simulink model "MPC_Demo_wuguzhang"  (R2024a)
settings: Solver=ode1  StartTime=0.001  StopTime=16  FixedStep=0.001  RelTol=1e-3  EnableMultiTasking=on
model workspace (MAT data in the model file):
  cc = 10
libraries: simulink x3, SignalEditorBlockLib x3, Solver_SF x1, slpidlib x1
(part 1 of 5)
settings Model: Creator=Dell  LastModifiedBy=Xiao Hu
settings SolverCC: AlgebraicLoopSolver=TrustRegion
settings OptimizationCC: LifeSpan=inf
settings DebuggingCC: MultiTaskRateTransMsg=warning  UnconnectedInputMsg=warning  UnconnectedOutputMsg=warning  UnconnectedLineMsg=warning  SFUnexpectedBacktrackingDiag=warning  SFNoUnconditionalDefaultTransitionDiag=warning  SFExecutionAtInitializationDiag=none  ArithmeticOperatorsInVariantConditions=warning
settings ModelReferenceCC: EnableRefExpFcnMdlSchedulingChecks=on
settings SFSimCC: SimUseLocalCustomCode=off  CustomCodeUndefinedFunction=UseInterfaceOnly
settings RTWCC: RTWUseLocalCustomCode=off  GPUComputeCapability=3.5
settings CodeAppCC: StateflowObjectComments=on
settings GRTTargetCC: TargetLangStandard=C89/C90 (ANSI)
settings ConfigComp: CovMetricSettings=dw  CovSaveCumulativeToWorkspaceVar=on  CovSaveSingleToWorkspaceVar=on  CovExternalEMLEnable=off

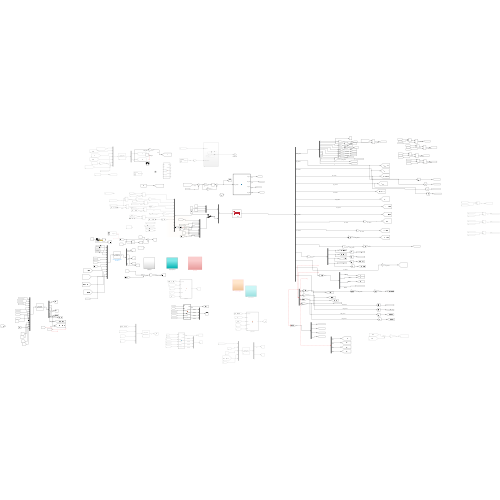
[thumbnail: Simulink's stored preview of the top-level diagram]
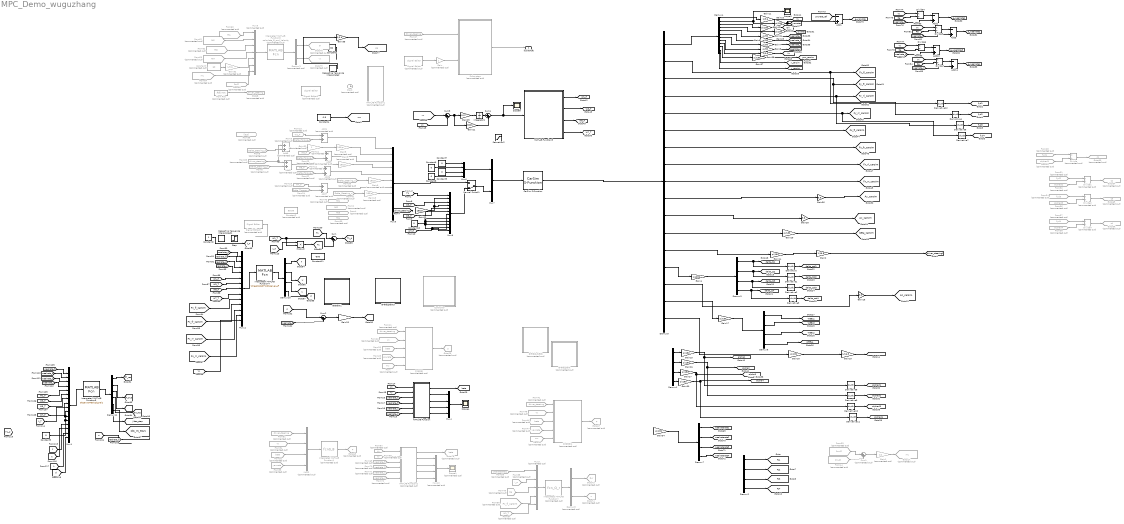
== system MPC_Demo_wuguzhang ==
  note: Product
  Add{1..3,10..11} (5 alike) : Sum  Inputs=-+
  Add{4..9} (6 alike) : Sum  Commented=on
  CarSim S-Function : Solver_SF/CarSim S-Function  Priority=1  SIMFILE=simfile.sim  Run_RTs=off  vs_state_ind=Run  StopMode_ind=Vehicle Model
  Clock : Clock  Commented=on
  Constant : Constant  Value=80
  Constant1 : Constant  Commented=on  Value=60
  Constant{5..10} (6 alike) : Constant  Value=0
  Constant11 : Constant  Value=-500
  Constant2 : Constant
  Constant3 : Constant  Commented=on  Value=89.99
  Constant4 : Constant  Value=0.8
  Controller : Subsystem  Commented=on
  Demux{1..3,6..7,10} (6 alike) : Demux
  Demux11 : Demux  Outputs=6
  Demux4 : Demux  Outputs=12
  Demux5 : Demux  Outputs=[12 1 1 1 1 1 1 1 1 1 1 1 1 4 1 4 1]
  Demux8 : Demux  Commented=on  Outputs=2
  Demux9 : Demux  Commented=on  Outputs=2
  Derivative{,1..4,6..12} (12 alike) : Derivative
  Divide{,1..3} (4 alike) : Product  Commented=on  Inputs=*/
  Divide{4..7} (4 alike) : Product  Inputs=*/
  From : From  Commented=on  GotoTag=mu  TagVisibility=global
  From File : FromFile  Commented=on  FileName=角度.mat  OutDataTypeStr=double  SampleTime=0.001
  From{11,27,41,51} (4 alike) : From  Commented=on  GotoTag=driver_steering  TagVisibility=global
  From12 : From  Commented=on  GotoTag=W5_T  TagVisibility=global
  From13 : From  Commented=on  GotoTag=W1_T  TagVisibility=global
  From2 : From  Commented=on  GotoTag=Fd2  TagVisibility=global
  From20 : From  Commented=on  GotoTag=beta  TagVisibility=global
  From21 : From  Commented=on  GotoTag=W3_T  TagVisibility=global
  From22 : From  Commented=on  GotoTag=Delta_Torque_rl  TagVisibility=global
  From23 : From  Commented=on  GotoTag=Delta_Torque_fr  TagVisibility=global
  From24 : From  Commented=on  GotoTag=Delta_Torque_rr  TagVisibility=global
  From25 : From  Commented=on  GotoTag=yawrate  TagVisibility=global
  From{26,48,54,67} (4 alike) : From  Commented=on  GotoTag=Vx  TagVisibility=global
  From28 : From  Commented=on  GotoTag=fyd1  TagVisibility=global
  From29 : From  Commented=on  GotoTag=W7_T  TagVisibility=global
  From3 : From  Commented=on  GotoTag=Delta_Torque_fl  TagVisibility=global
  From30 : From  Commented=on  GotoTag=alphad1  TagVisibility=global
  From31 : From  Commented=on  GotoTag=fyd2  TagVisibility=global
  From32 : From  Commented=on  GotoTag=alphad2  TagVisibility=global
  From33 : From  Commented=on  GotoTag=mu1  TagVisibility=global
  From34 : From  Commented=on  GotoTag=fyd3  TagVisibility=global
  From35 : From  Commented=on  GotoTag=driver_steering
  From36 : From  Commented=on  GotoTag=alphad3  TagVisibility=global
  From37 : From  Commented=on  GotoTag=fyd4  TagVisibility=global
  From38 : From  Commented=on  GotoTag=alphad4  TagVisibility=global
  From39 : From  Commented=on  GotoTag=Delta_Steering_rl  TagVisibility=global
  From4 : From  Commented=on  GotoTag=Fd3  TagVisibility=global
  From40 : From  Commented=on  GotoTag=mu  TagVisibility=global
  From42 : From  Commented=on  GotoTag=Delta_Steering_rr  TagVisibility=global
  From43 : From  Commented=on  GotoTag=Fd1  TagVisibility=global
  From44 : From  Commented=on  GotoTag=mu2  TagVisibility=global
  From46 : From  Commented=on  GotoTag=beta  TagVisibility=global
  From47 : From  Commented=on  GotoTag=yawrate  TagVisibility=global
  From49 : From  Commented=on  GotoTag=Re  TagVisibility=global
  From5 : From  Commented=on  GotoTag=Delta_Steering_fl  TagVisibility=global
  From50 : From  Commented=on  GotoTag=Fd4  TagVisibility=global
  From52 : From  Commented=on  GotoTag=beta  TagVisibility=global
  From53 : From  Commented=on  GotoTag=yawrate  TagVisibility=global
  From55 : From  Commented=on  GotoTag=I_w  TagVisibility=global
  From56 : From  Commented=on  GotoTag=Fx_fl_carsim  TagVisibility=global
  From57 : From  Commented=on  GotoTag=W1_T  TagVisibility=global
  From58 : From  Commented=on  GotoTag=last
  From59 : From  Commented=on  GotoTag=weelraterate1  TagVisibility=global
  From6 : From  Commented=on  GotoTag=Delta_Steering_fr  TagVisibility=global
  From60 : From  Commented=on  GotoTag=Fz1  TagVisibility=global
  From61 : From  Commented=on  GotoTag=Fz2  TagVisibility=global
  From62 : From  Commented=on  GotoTag=Fz3  TagVisibility=global
  From63 : From  Commented=on  GotoTag=Fz4  TagVisibility=global
  From64 : From  Commented=on  GotoTag=mu  TagVisibility=global
  From66 : From  Commented=on  GotoTag=tw1  TagVisibility=global
  From68 : From  Commented=on  GotoTag=Vy  TagVisibility=global
  From69 : From  Commented=on  GotoTag=weelrate_fl  TagVisibility=global
  From70 : From  Commented=on  GotoTag=weelrate_fr  TagVisibility=global
  From71 : From  Commented=on  GotoTag=weelrate_rl  TagVisibility=global
  From72 : From  Commented=on  GotoTag=weelrate_rr  TagVisibility=global
  Gain : Gain  Commented=on
  Gain1 : Gain  Commented=on  Gain=1/2
  Gain{10,12,14..15,17..18,23,26..27,29..30,34,37} (13 alike) : Gain  Gain=pi/180
  Gain11 : Gain  Gain=1/3.6
  Gain{3,5,9,13} (4 alike) : Gain  Commented=on  Gain=180/pi
  Gain16 : Gain  Gain=9.8
  Gain19 : Gain  Gain=1/16.8
  Gain2 : Gain  Gain=1/16.8
  Gain20 : Gain  Gain=1.5/0.005
  Gain21 : Gain  Gain=5000
  Gain22 : Gain  Gain=180/pi
  Gain{6..8,24} (4 alike) : Gain  Gain=pi/30
  Gain25 : Gain  Gain=0.07
  Gain28 : Gain  Gain=9.8
  Gain32 : Gain  Commented=on  Gain=1/3.6
  Gain35 : Gain  Gain=1/3.6
  Gain36 : Gain  Gain=9.8
  Gain38 : Gain  Gain=1/3.6
  Gain39 : Gain  Commented=on
  Gain4 : Gain  Gain=1/1000
  Goto17 : Goto  Commented=on  GotoTag=mu  TagVisibility=global
  Goto28 : Goto  Commented=on  GotoTag=p  TagVisibility=global
  Goto59 : Goto  Commented=on  GotoTag=c1  TagVisibility=global
  Goto64 : Goto  Commented=on  GotoTag=c2  TagVisibility=global
  Goto65 : Goto  Commented=on  GotoTag=c3  TagVisibility=global
  Goto66 : Goto  Commented=on  GotoTag=c4  TagVisibility=global
  Goto67 : Goto  Commented=on  GotoTag=p  TagVisibility=global
  Goto68 : Goto  Commented=on  GotoTag=p  TagVisibility=global
  Goto73 : Goto  Commented=on  GotoTag=Q_r  TagVisibility=global
  Goto74 : Goto  Commented=on  GotoTag=n  TagVisibility=global
  Goto75 : Goto  Commented=on  GotoTag=vx  TagVisibility=global
  Goto76 : Goto  Commented=on  GotoTag=G  TagVisibility=global
  Goto78 : Goto  Commented=on  GotoTag=beta  TagVisibility=global
  Goto8 : Goto  Commented=on  GotoTag=driver_steering  TagVisibility=global
  Integrator1 : Integrator
  Interpreted MATLAB Function1 : MATLABFcn  Commented=on  MATLABFcn=fcn0_8  OutputDimensions=1  Output1D=off
  Interpreted MATLAB Function2 : MATLABFcn  Commented=on  MATLABFcn=fcn_Q_r  OutputDimensions=2  Output1D=off
  Interpreted MATLAB Function3 : MATLABFcn  Commented=on  MATLABFcn=calculate_G_and_Velocity  OutputDimensions=2  Output1D=off
  Interpreted MATLAB Function4 : MATLABFcn  MATLABFcn=WheelRotASTWObserver_LF  OutputDimensions=4  Output1D=off
  Interpreted MATLAB Function5 : MATLABFcn  MATLABFcn=ObserverMetricSignals  OutputDimensions=6  Output1D=off
  MATLAB Function : MATLAB Function  TreatAsAtomicUnit=on
  MATLAB Function1 : MATLAB Function  Commented=on  TreatAsAtomicUnit=on
  MATLAB Function2 : MATLAB Function  Commented=on  TreatAsAtomicUnit=on
  MATLAB Function5 : MATLAB Function  TreatAsAtomicUnit=on
  Manual Switch1 : ManualSwitch  CurrentSetting=0
  Mux1 : Mux  Inputs=16
  Mux10 : Mux  Commented=on
  Mux11 : Mux  Inputs=13
  Mux2 : Mux  Commented=on
  Mux3 : Mux  Commented=on  Inputs=5
  Mux4 : Mux
  Mux5 : Mux  Inputs=12
  Mux6 : Mux
  Mux7 : Mux  Inputs=[4,12]
  Mux8 : Mux  Inputs=12
  Mux9 : Mux  Commented=on  Inputs=7
  Product : Product
  Repeating Sequence Interpolated : simulink/Sources/Repeating Sequence Interpolated  OutValues=[60.76 83.52 41].'  TimeValues=[0 8.5 16].'  LookUpMeth=Interpolation-Use End Values  tsamp=0.001  OutMin=[]  OutMax=[]  OutDataTypeStr=double  OutputDataTypeScalingMode=double  OutDataType=fixdt(0,8)  OutScaling=2^-10
  Repeating Sequence Interpolated1 : simulink/Sources/Repeating Sequence Interpolated  OutValues=[1 1 0.2 0.2].'  TimeValues=[0 3 3.01 16].'  LookUpMeth=Interpolation-Use End Values  tsamp=0.001  OutMin=[]  OutMax=[]  OutDataTypeStr=double  OutputDataTypeScalingMode=double  OutDataType=fixdt(0,8)  OutScaling=2^-10
  Saturation2 : Saturate  UpperLimit=6400  LowerLimit=-6400
  Scope1 : Scope  Commented=on
  Scope3 : Scope
  Scope4 : Scope
  Scope8 : Scope
  Signal Editor : SignalEditorBlockLib/Signal Editor  Commented=on  FileName=Tdist.mat  ActiveScenario=Scenario  ActiveSignal=Signal 1  IsBus=off  OutputBusObjectStr=Bus: BusObject  SampleTime=0  Interpolate=off  ZeroCross=off  OutputAfterFinalValue=Setting to zero  Unit=inherit  PreserveSignalName=on  ApplySigPropsToAllScenarios=on  ApplySigPropsToAllSignals=off
  Signal Editor1 : SignalEditorBlockLib/Signal Editor  Commented=on  FileName=untitled111.mat  ActiveScenario=Scenario  ActiveSignal=Signal 1  IsBus=off  OutputBusObjectStr=Bus: BusObject  SampleTime=0  Interpolate=off  ZeroCross=off  OutputAfterFinalValue=Holding final value  Unit=inherit  PreserveSignalName=on  ApplySigPropsToAllScenarios=on  ApplySigPropsToAllSignals=off
  Signal Editor2 : SignalEditorBlockLib/Signal Editor  Commented=on  FileName=Tdist.mat  ActiveScenario=Scenario  ActiveSignal=Signal 1  IsBus=off  OutputBusObjectStr=Bus: BusObject  SampleTime=0  Interpolate=off  ZeroCross=off  OutputAfterFinalValue=Setting to zero  Unit=inherit  PreserveSignalName=on  ApplySigPropsToAllScenarios=on  ApplySigPropsToAllSignals=off
  Step : Step  Time=4  Before=1  After=-1  SampleTime=0
  Subsystem : Subsystem  Commented=on
  Sum : Sum  Inputs=|+-
  Sum1 : Sum  Commented=on  Inputs=|++
  Sum2 : Sum  Inputs=|-+
  Sum3 : Sum  Inputs=|+-
  Sum4 : Sum  Inputs=|++
  区域判断 : MATLAB Function  Commented=on  TreatAsAtomicUnit=on
  区域判断1 : MATLAB Function  Commented=on  TreatAsAtomicUnit=on
  参数模块1 : Subsystem
  参考值生成模块 : Subsystem  Commented=on
  参考模型模块 : Subsystem  Commented=on
  参考模型模块3 : Subsystem
  实际转向角 : Outport
  tag scope: Ax_carsim=global, Ay_carsim=global, Az_carsim=global, Fx_fl_carsim=global, Fx_fr_carsim=global, Fx_rl_carsim=global, Fx_rr_carsim=global, Fy_fl_carsim=global, Fy_fr_carsim=global, Fy_rl_carsim=global, Fy_rr_carsim=global, Fz1=global, Fz2=global, Fz3=global, Fz4=global, T1=global, T1_d=global, Vx=global, Vy=global, W1_T=global, W3_T=global, W5_T=global, W7_T=global, WEEL1=global, WEEL2=global, WEEL3=global, WEEL4=global, alpha1=global, alpha2=global, alpha3=global, alpha4=global, alphad1=global, alphad2=global, alphad3=global, alphad4=global, beta=global, beta_carsim=global, d=global, d_model=global, delta_zs1=global, delta_zs2=global, delta_zs3=global, delta_zs4=global, delta_zsd1=global, delta_zsd2=global, delta_zsd3=global, delta_zsd4=global, driver_steering10=global, driver_steering5=global, e_weelrate1=global, e_weelrate2=global, e_weelrate3=global, e_weelrate4=global, e_yawrate=global, err_res=global, err_true=global, f=global, fT_res=global, fT_true=global, fyd1=global, fyd2=global, fyd3=global, fyd4=global, jitter_step=global, k=global, k_T=global, mu=global, obs_inj_equiv=global, roll=global, rollrate=global, vx=global, w=global, weelrate_fl=global, weelrate_fr=global, weelrate_rl=global, weelrate_rr=global, weelraterate1=global, weelraterate2=global, weelraterate3=global, weelraterate4=global, x_carsim=global, y_carsim=global, yaw_carsim=global, yawrate=global
  wires:
  [Vx] -> MATLAB Function/1(Vx)
  [Vy] -> MATLAB Function/2(Vy)
  [weelrate_fl] -> MATLAB Function/3(omega_1)
  [weelrate_fr] -> MATLAB Function/4(omega_2)
  [weelrate_rl] -> MATLAB Function/5(omega_3)
  [weelrate_rr] -> MATLAB Function/6(omega_4)
  MATLAB Function/2(lamda1) -> Mux4/1  "lamda1"
  MATLAB Function/3(lamda2) -> Mux4/2  "lamda2"
  MATLAB Function/4(lamda3) -> Mux4/3  "lamda3"
  MATLAB Function/5(lamda4) -> Mux4/4  "lamda4"
  Mux4/1 -> Scope4/1
  MATLAB Function/1(beta) -> [beta]  "beta"
  Gain23/1 -> [rollrate]  "rollrate"
  Demux4/2 -> Scope3/1, Gain10/1
  Gain36/1 -> [Ay_carsim]  "Ay_carsim"
  Demux5/4 -> Derivative6/1, [Fy_rl_carsim]  "Fyrl_carsim"
  Demux4/8 -> Gain8/1
  Demux5/8 -> [Fx_rl_carsim]  "Fzrl_carsim"
  Demux4/12 -> [y_carsim]  "Y"
  Gain28/1 -> [Ax_carsim]  "Ax_carsim"
  Gain29/1 -> [beta_carsim]  "beta_carsim"
  Demux4/10 -> Gain37/1
  Gain37/1 -> [yaw_carsim]  "yaw_carsim"
  Demux4/9 -> Gain38/1
  Gain38/1 -> [Vx]  "vx_carsim"
  Demux5/1 -> Demux4/1  "delta_carsim"
  Demux5/3 -> Derivative4/1, [Fy_fr_carsim]  "Fyfr_carsim"
  Demux4/3 -> Gain12/1
  Demux4/1 -> Gain11/1
  Gain12/1 -> [roll]  "roll"
  Gain10/1 -> Add1/2, [yawrate]  "yawrate"
  Gain8/1 -> [weelrate_rr]  "weelrate4"
  Demux5/9 -> [Fx_rr_carsim]  "Fzrr_carsim"
  Gain11/1 -> [Vy]  "Vy"
  Demux4/5 -> Gain24/1
  Demux4/6 -> Gain6/1
  Gain7/1 -> [weelrate_rl]  "weelrate3"
  Gain6/1 -> [weelrate_fr]  "weelrate2"
  Gain24/1 -> [weelrate_fl]  "轮速实际值"
  Demux5/11 -> Gain28/1  "w_rl_carsim"
  Demux4/4 -> Gain23/1
  Demux5/5 -> Derivative7/1, [Fy_rr_carsim]  "Fyrr_carsim"
  Demux4/7 -> Gain7/1
  Demux5/2 -> Derivative12/1, [Fy_fl_carsim]  "Fyfl_carsim"
  Demux5/6 -> [Fx_fl_carsim]  "Fzfl_carsim"
  Demux5/10 -> Gain36/1  "Ay_carsim"
  Demux4/11 -> [x_carsim]  "X"
  Demux5/12 -> Gain29/1
  Demux5/7 -> [Fx_fr_carsim]  "Fzfr_carsim"
  CarSim S-Function/1 -> Demux5/1
  Demux5/13 -> Gain14/1
  Gain2/1 -> [driver_steering5]  "ds"
  ? -> Demux2/1
  Demux2/1 -> [Fz1]  "mu1"
  Demux2/2 -> [Fz2]  "mu2"
  Demux2/3 -> [Fz3]  "mu3"
  Demux2/4 -> [Fz4]  "mu4"
  From33/1 -> Sum1/1
  From44/1 -> Sum1/2
  Sum1/1 -> Gain1/1
  Gain1/1 -> Goto17/1  "ds"
  Constant4/1 -> [mu]
  Demux5/14 -> Gain4/1
  Demux3/1 -> Derivative/1, [delta_zs1]
  Demux3/2 -> Derivative1/1, [delta_zs2]
  Demux3/3 -> Derivative2/1, [delta_zs3]
  Demux3/4 -> Derivative3/1, [delta_zs4]
  Derivative/1 -> [delta_zsd1]
  Derivative1/1 -> [delta_zsd2]
  Derivative2/1 -> [delta_zsd3]
  Derivative3/1 -> [delta_zsd4]
  Gain4/1 -> Demux3/1
  Gain21/1 -> Sum4/2
  MATLAB Function5/2(Tor_R1) -> [W3_T]  "T_R1"
  Sum3/1 -> Gain25/1, Gain21/1
  Sum4/1 -> Scope8/1, MATLAB Function5/1(Drive_torque)
  MATLAB Function5/4(Tor_R2) -> [W7_T]  "T_R2"
  [vx] -> Sum3/1  "Vx_d"
  Integrator1/1 -> Sum4/1
  Gain25/1 -> Integrator1/1
  [Vx] -> Sum3/2  "vx"
  MATLAB Function5/1(Tor_L1) -> [W1_T]  "T_L1"
  MATLAB Function5/3(Tor_L2) -> [W5_T]  "T_L2"
  From6/1 -> Add8/2  "delta3"
  From39/1 -> Gain9/1
  From5/1 -> Add9/2
  Add8/1 -> Gain3/1  "总的转角2"
  Constant7/1 -> Mux6/1
  Constant9/1 -> Mux6/3
  From35/1 -> Add9/1, Add8/1
  Add6/1 -> Mux5/5  "T3"
  Mux8/1 -> Manual Switch1/2  "u"
  From22/1 -> Add6/2  "delta3"
  Mux7/1 -> CarSim S-Function/1  "u"
  From13/1 -> Add4/1
  Constant6/1 -> Mux6/2
  From23/1 -> Add5/2  "delta2"
  From24/1 -> Add7/2
  From3/1 -> Add4/2  "delta1"
  [driver_steering] -> ?
  Mux5/1 -> Manual Switch1/1  "u"
  Mux6/1 -> Mux7/1  "u"
  Constant8/1 -> Mux6/4
  From21/1 -> Add5/1
  From29/1 -> Add7/1  "delta4"
  [W7_T] -> Mux8/7  "q1"
  [W3_T] -> Mux8/3  "q1"
  Constant10/1 -> Mux8/12, Mux8/11, Mux8/10, Mux8/6, Mux8/8, Mux8/9
  From File/1 -> Goto8/1
  From12/1 -> Add6/1
  From42/1 -> Gain13/1
  Gain14/1 -> Gain2/1  "beta_carsim"
  Demux5/15 -> Gain16/1  "w_rl_carsim"
  Gain16/1 -> [Az_carsim]  "Ax_carsim"
  Demux6/2 -> [WEEL3]  "WEEL3"
  Demux6/4 -> [WEEL4]  "WEEL4"
  Demux6/3 -> [WEEL2]  "WEEL2"
  Demux5/16 -> Gain17/1
  Demux6/1 -> [WEEL1]  "WEEL1"
  Gain17/1 -> Demux6/1
  Manual Switch1/1 -> Mux7/2  "add_Mz"
  Demux5/17 -> Gain18/1
  Gain18/1 -> Gain19/1  "beta_carsim"
  Gain19/1 -> [driver_steering10]  "ds1"
  From11/1 -> 区域判断/1(sw_angle)
  区域判断/1(p) -> Goto28/1  "p"
  From26/1 -> 区域判断/2(Vx)
  From/1 -> 区域判断/5(miu)
  From25/1 -> 区域判断/4(gamma)
  From20/1 -> 区域判断/3(beta)
  Subsystem/1(实际转向角) -> 实际转向角/1
  Gain/1 -> Subsystem/2(外部扰动力矩)
  Signal Editor/1 -> Gain/1  "Tdist"
  From27/1 -> Subsystem/1(期望转向)
  Signal Editor2/1 -> ?  "Tdist"
  Gain22/1 -> Mux8/2, Mux8/4
  Derivative7/1 -> [fyd4]
  Derivative6/1 -> [fyd3]
  Derivative12/1 -> [fyd1]
  Demux1/1 -> Gain15/1  "Fyfl_carsim"
  Derivative11/1 -> [alphad4]
  Demux1/4 -> Gain30/1  "Fyrr_carsim"
  Derivative8/1 -> [alphad1]
  Demux1/3 -> Gain27/1  "Fyrl_carsim"
  Derivative9/1 -> [alphad2]
  Demux1/2 -> Gain26/1  "Fyfr_carsim"
  Derivative10/1 -> [alphad3]
  ? -> Demux1/1
  From28/1 -> Divide/1
  From30/1 -> Divide/2
  Divide/1 -> Goto59/1  "c1"
  From31/1 -> Divide1/1
  Divide1/1 -> Goto64/1  "c2"
  From32/1 -> Divide1/2
  From34/1 -> Divide2/1
  Divide2/1 -> Goto65/1  "c3"
  From36/1 -> Divide2/2
  From38/1 -> Divide3/2
  Divide3/1 -> Goto66/1
  From37/1 -> Divide3/1
  Gain15/1 -> Derivative8/1, [alpha1]  "beta_carsim"
  Gain26/1 -> Derivative9/1, [alpha2]  "beta_carsim"
  Gain27/1 -> Derivative10/1, [alpha3]  "beta_carsim"
  Gain30/1 -> Derivative11/1, [alpha4]  "beta_carsim"
  Derivative4/1 -> [fyd2]
  From48/1 -> 区域判断1/2(Vx)
  区域判断1/1(p) -> Goto67/1  "p"
  From46/1 -> 区域判断1/3(beta)
  From41/1 -> 区域判断1/1(sw_angle)
  From47/1 -> 区域判断1/4(gamma)
  From40/1 -> 区域判断1/5(miu)
  From54/1 -> Mux2/2
  From52/1 -> Mux2/3
  From51/1 -> Mux2/1
  From53/1 -> Mux2/4
  Mux2/1 -> Interpreted MATLAB Function1/1
  Interpreted MATLAB Function1/1 -> Goto68/1  "p"
  Gain5/1 -> Mux5/2
  Add5/1 -> Mux5/3  "T2"
  Gain3/1 -> Mux5/4
  Gain9/1 -> Mux5/6
  Add7/1 -> Mux5/7  "T4"
  Gain13/1 -> Mux5/8
  Demux7/3 -> [weelraterate3]
  Demux7/1 -> [weelraterate1]
  Demux7/2 -> [weelraterate2]
  Demux7/4 -> [weelraterate4]
  Gain34/1 -> Demux7/1
  ? -> Gain34/1
  From59/1 -> Mux3/1
  From55/1 -> Mux3/2
  From49/1 -> Mux3/3
  From56/1 -> Mux3/4
  Mux3/1 -> Interpreted MATLAB Function2/1
  From57/1 -> Mux3/5
  Demux8/1 -> Goto73/1  "Q_r"
  Interpreted MATLAB Function2/1 -> Demux8/1
  Demux8/2 -> Goto74/1  "n"
  From62/1 -> Mux9/3
  From63/1 -> Mux9/4
  From60/1 -> Mux9/1
  Mux9/1 -> Interpreted MATLAB Function3/1
  From61/1 -> Mux9/2
  Constant1/1 -> Gain32/1
  Interpreted MATLAB Function3/1 -> Demux9/1  "p"
  Demux9/2 -> Goto75/1  "vx"
  Demux9/1 -> Goto76/1
  From64/1 -> Mux9/6  "Vx_d"
  Gain32/1 -> Mux9/5  "Vx_d"
  From66/1 -> Mux9/7
  Gain35/1 -> [vx]  "vx_d"
  Repeating Sequence Interpolated/1 -> Gain35/1  "theta_des"
  From72/1 -> MATLAB Function2/6(omega_4)
  MATLAB Function2/2(lamda1) -> Mux10/1  "lamda1"
  MATLAB Function2/3(lamda2) -> Mux10/2  "lamda2"
  MATLAB Function2/5(lamda4) -> Mux10/4  "lamda4"
  From71/1 -> MATLAB Function2/5(omega_3)
  MATLAB Function2/4(lamda3) -> Mux10/3  "lamda3"
  From70/1 -> MATLAB Function2/4(omega_2)
  MATLAB Function2/1(beta) -> Goto78/1  "beta"
  Mux10/1 -> Scope1/1
  From68/1 -> MATLAB Function2/2(Vy)
  From67/1 -> MATLAB Function2/1(Vx)
  From69/1 -> MATLAB Function2/3(omega_1)
  [yawrate_ref] -> Add1/1
  Add1/1 -> [e_yawrate]  "e_yawrate"
  [Vx] -> Divide4/1
  [Re] -> Divide4/2
  Divide4/1 -> Add2/1  "c1"
  [weelrate_fl] -> Add2/2
  Divide5/1 -> Add3/1  "c1"
  [Re] -> Divide5/2
  [weelrate_fr] -> Add3/2
  [Vx] -> Divide5/1
  [Re] -> Divide6/2
  [Vx] -> Divide6/1
  [weelrate_rr] -> Add11/2
  Divide7/1 -> Add11/1  "c1"
  Divide6/1 -> Add10/1  "c1"
  [Re] -> Divide7/2
  [Vx] -> Divide7/1
  [weelrate_rl] -> Add10/2
  Add2/1 -> [e_weelrate1]  "e_weelrate1"
  Add3/1 -> [e_weelrate2]  "e_weelrate2"
  Add10/1 -> [e_weelrate3]  "e_weelrate3"
  Add11/1 -> [e_weelrate4]  "e_weelrate4"
  Add4/1 -> Mux5/1  "T1"
  Add9/1 -> Gain39/1  "总的转角1"
  Gain39/1 -> Gain5/1
  Mux11/1 -> Interpreted MATLAB Function4/1
  [weelrate_fl] -> Mux11/1
  [weelrate_fr] -> Mux11/2
  [weelrate_rl] -> Mux11/3
  [weelrate_rr] -> Mux11/4
  [W1_T] -> Mux11/5
  [W3_T] -> Mux11/6
  [W5_T] -> Mux11/7
  [W7_T] -> Mux11/8
  [Fx_fl_carsim] -> Mux11/9
  [Fx_fr_carsim] -> Mux11/10
  [Fx_rr_carsim] -> Mux11/11
  [Fx_rr_carsim] -> Mux11/12
  Interpreted MATLAB Function4/1 -> Demux10/1  "p"
  Demux10/3 -> [k]  "k"
  Demux10/2 -> [w]  "轮速估计值"
  Demux10/4 -> [d]  "d"
  Demux10/1 -> [f]  "未知输入估计值"
  [Vx] -> Mux11/13
  [T1] -> Mux8/1
  [W1_T] -> Sum/2, Product/2
  Product/1 -> [T1]
  [T1] -> Sum/1
  Sum/1 -> [T1_d]
  Sum2/1 -> Gain20/1  "d_model"
  [w] -> Sum2/1
  [weelrate_fl] -> Sum2/2
  Gain20/1 -> [d_model]  "未知输入实际值"
  [W5_T] -> Mux8/5
  Constant2/1 -> [k_T]
  [w] -> ?
  [weelrate_fl] -> ?
  Demux11/4 -> [err_res]  "err_res"
  Demux11/1 -> [fT_res]  "fT_res"
  [W5_T] -> Mux1/7
  Interpreted MATLAB Function5/1 -> Demux11/1  "p"
  Mux1/1 -> Interpreted MATLAB Function5/1
  [W7_T] -> Mux1/8
  [W1_T] -> Mux1/5
  [weelrate_fr] -> Mux1/2
  [weelrate_rr] -> Mux1/4
  Demux11/3 -> [err_true]  "err_true"
  [W3_T] -> Mux1/6
  [weelrate_rl] -> Mux1/3
  [weelrate_fl] -> Mux1/1
  Demux11/2 -> [fT_true]  "fT_true"
  [k_T] -> Product/1
  [k_T] -> Mux1/9
  Constant5/1 -> Mux1/11, Mux1/10, Mux1/12
  [f] -> Mux1/13
  [w] -> Mux1/14
  [k] -> Mux1/15
  [d] -> Mux1/16
  Demux11/5 -> [jitter_step]  "jitter_step"
  Demux11/6 -> [obs_inj_equiv]  "obs_inj_equiv"
  Constant/1 -> ?  "theta_des"

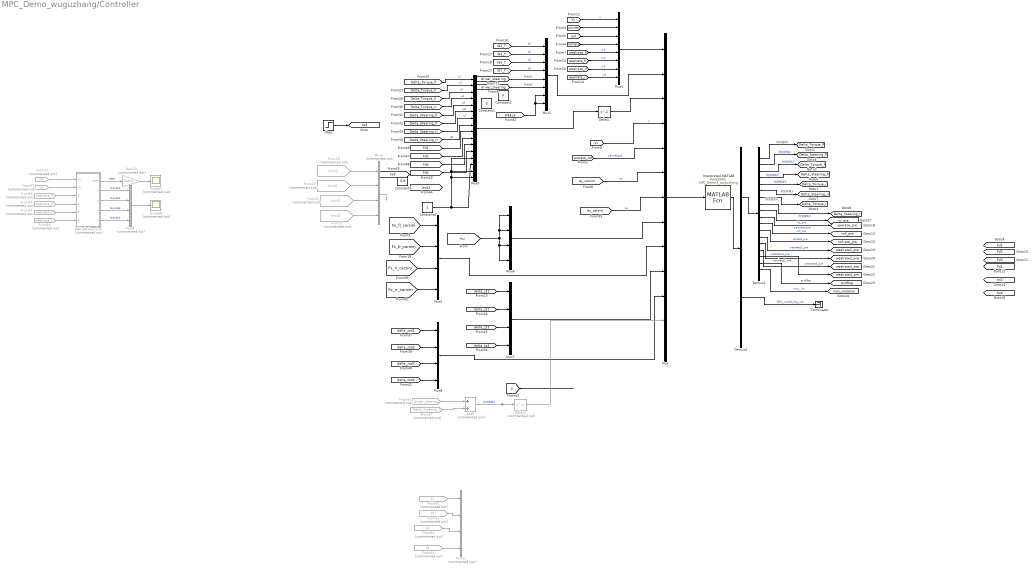
== system MPC_Demo_wuguzhang/Controller ==
  Add9 : Sum  Commented=on
  Constant1 : Constant  Value=0
  Constant2 : Constant  Value=0
  Constant3 : Constant  Value=0.8
  Constant4 : Constant
  Delay1 : Delay  DelayLength=1  InitialCondition=0
  Delay2 : Delay  Commented=on  DelayLength=1  InitialCondition=0
  Demux1 : Demux  Outputs=18
  Demux2 : Demux  Outputs=[18,481]
  From19 : From  Commented=on  GotoTag=mu1  TagVisibility=global
  From20 : From  Commented=on  GotoTag=mu2  TagVisibility=global
  From21 : From  Commented=on  GotoTag=mu3  TagVisibility=global
  From22 : From  Commented=on  GotoTag=mu4  TagVisibility=global
  From50 : From  Commented=on  GotoTag=driver_steering  TagVisibility=global
  From51 : From  Commented=on  GotoTag=Vx  TagVisibility=global
  From52 : From  Commented=on  GotoTag=Vy  TagVisibility=global
  From53 : From  Commented=on  GotoTag=weelrate_fl  TagVisibility=global
  From54 : From  Commented=on  GotoTag=weelrate_fr  TagVisibility=global
  From55 : From  Commented=on  GotoTag=weelrate_rl  TagVisibility=global
  From56 : From  Commented=on  GotoTag=weelrate_rr  TagVisibility=global
  From57 : From  Commented=on  GotoTag=Delta_Steering_fl  TagVisibility=global
  From60 : From  Commented=on  GotoTag=c1  TagVisibility=global
  From61 : From  Commented=on  GotoTag=c2  TagVisibility=global
  From62 : From  Commented=on  GotoTag=c3  TagVisibility=global
  From63 : From  Commented=on  GotoTag=c4  TagVisibility=global
  Gain15 : Gain  Commented=on  Gain=180/pi
  Interpreted MATLAB Function1 : MATLABFcn  MATLABFcn=MPC_Demo3_wuguzhang  OutputDimensions=499  Output1D=off
  MATLAB Function : MATLAB Function  Commented=on  TreatAsAtomicUnit=on
  Mux : Mux  Inputs=[8,8,16,1,1,1,1,4,4,4,4,1,1]
  Mux1 : Mux  Inputs=8
  Mux12 : Mux  Commented=on
  Mux2 : Mux  Inputs=8
  Mux3 : Mux  Inputs=16
  Mux4 : Mux  Commented=on
  Mux{5..8} (4 alike) : Mux
  Mux9 : Mux  Commented=on
  Scope1 : Scope  Commented=on
  Scope4 : Scope  Commented=on
  Step : Step  Time=3  Before=1  After=0  SampleTime=0
  Terminator : Terminator
  tag scope: Delta_Steering_fl=global, Delta_Steering_fr=global, Delta_Steering_rl=global, Delta_Steering_rr=global, Delta_Torque_fl=global, Delta_Torque_fr=global, Delta_Torque_rl=global, Delta_Torque_rr=global, Fd1=global, Fd2=global, Fd3=global, Fd4=global, exitflag=global, max_violation=global, roll_pre=global, rollrate_pre=global, tw2=global, tw3=global, tw4=global, vy_pre=global, weelrate1_pre=global, weelrate2_pre=global, weelrate3_pre=global, weelrate4_pre=global, yawrate_pre=global
  wires:
  [Vy] -> Mux1/1  "v"
  [yawrate] -> Mux1/2
  [roll] -> Mux1/3
  [rollrate] -> Mux1/4
  [weelrate_fl] -> Mux1/5  "w1"
  [weelrate_fr] -> Mux1/6  "w2"
  [weelrate_rl] -> Mux1/7  "w3"
  [weelrate_rr] -> Mux1/8  "w4"
  [W7_T] -> Mux2/4  "q4"
  [W5_T] -> Mux2/3  "q3"
  [W3_T] -> Mux2/2  "q2"
  [W1_T] -> Mux2/1  "q1"
  [Delta_Steering_fl] -> Mux3/5  "u5"
  [Delta_Steering_rl] -> Mux3/7  "u7"
  [Delta_Torque_rr] -> Mux3/4  "u4"
  [Delta_Torque_fr] -> Mux3/2  "u2"
  [Delta_Steering_fr] -> Mux3/6  "u6"
  [Delta_Torque_fl] -> Mux3/1  "u1"
  [Delta_Steering_rr] -> Mux3/8  "u8"
  [Delta_Torque_rl] -> Mux3/3  "u3"
  Mux3/1 -> Delay1/1
  Interpreted MATLAB Function1/1 -> Demux2/1
  Demux1/8 -> [Delta_Steering_rr]  "附加转角4"
  Demux1/1 -> [Delta_Torque_fl]  "附加扭矩1"
  Mux1/1 -> Mux/1
  Mux2/1 -> Mux/2
  Delay1/1 -> Mux/3
  [Vx] -> Mux/4  "u"
  Demux1/2 -> [Delta_Steering_fl]  "附加转角1"
  Demux1/4 -> [Delta_Steering_fr]  "附加转角2"
  Demux1/5 -> [Delta_Torque_rl]  "附加扭矩3"
  Demux1/6 -> [Delta_Steering_rl]  "附加转角3"
  Demux1/7 -> [Delta_Torque_rr]  "附加扭矩4"
  Mux/1 -> Interpreted MATLAB Function1/1
  [yawrate_ref] -> Mux/5  "yawrate_d"
  [Ay_carsim] -> Mux/6  "ay"
  [Ax_carsim] -> Mux/7  "ax"
  Mux4/1 -> ?
  [driver_steering] -> Mux2/6  "theta2"
  [Fx_fl_carsim] -> Mux5/1
  [Fx_fr_carsim] -> Mux5/2
  [Fx_rl_carsim] -> Mux5/3
  [Fx_rr_carsim] -> Mux5/4
  Mux5/1 -> Mux/9
  From19/1 -> Mux4/1
  From20/1 -> Mux4/2
  From21/1 -> Mux4/3
  From22/1 -> Mux4/4
  [mu] -> Mux6/2, Mux6/1, Mux6/4, Mux6/3
  Mux6/1 -> Mux/8
  Mux7/1 -> Mux/10
  [delta_zs1] -> Mux7/1
  [delta_zs2] -> Mux7/2
  [delta_zs3] -> Mux7/3
  [delta_zs4] -> Mux7/4
  [delta_zsd4] -> Mux8/4
  [delta_zsd2] -> Mux8/2
  [delta_zsd1] -> Mux8/1
  [delta_zsd3] -> Mux8/3
  Mux8/1 -> Mux/11
  ? -> [Fd1]  "fd1"
  ? -> [Fd2]  "fd2"
  ? -> [Fd3]  "fd3"
  ? -> [Fd4]  "fd4"
  [Fd4] -> Mux3/12
  [Fd3] -> Mux3/11
  [Fd2] -> Mux3/10
  [Fd1] -> Mux3/9
  Demux1/3 -> [Delta_Torque_fr]  "附加扭矩2"
  ? -> ?
  ? -> [tw2]
  ? -> ?
  ? -> [tw4]
  Constant4/1 -> Mux3/16, Mux3/15, Mux3/13, Mux3/14
  MATLAB Function/2(lamda1) -> Mux9/1  "lamda1"
  From56/1 -> MATLAB Function/6(omega_4)
  From53/1 -> MATLAB Function/3(omega_1)
  MATLAB Function/1(beta) -> Gain15/1  "beta"
  MATLAB Function/5(lamda4) -> Mux9/4  "lamda4"
  From51/1 -> MATLAB Function/1(Vx)
  From52/1 -> MATLAB Function/2(Vy)
  Mux9/1 -> Scope4/1
  From55/1 -> MATLAB Function/5(omega_3)
  MATLAB Function/4(lamda3) -> Mux9/3  "lamda3"
  MATLAB Function/3(lamda2) -> Mux9/2  "lamda2"
  From54/1 -> MATLAB Function/4(omega_2)
  Gain15/1 -> Scope1/1
  From60/1 -> Mux12/1
  From61/1 -> Mux12/2
  From62/1 -> Mux12/3
  From63/1 -> Mux12/4
  [p] -> ?
  Demux1/9 -> [vy_pre]  "Vy_pre"
  Add9/1 -> Delay2/1  "总的转角1"
  From57/1 -> Add9/2
  From50/1 -> Add9/1
  Delay2/1 -> Mux/12
  Demux1/10 -> [yawrate_pre]  "yawrate_pre"
  Step/1 -> [tw3]
  [WEEL3] -> Mux2/8, Mux2/7
  Demux1/11 -> [roll_pre]  "roll_pre"
  Demux1/12 -> [rollrate_pre]  "rollrate_pre"
  Demux1/13 -> [weelrate1_pre]  "weelrate1_pre"
  Demux1/14 -> [weelrate2_pre]  "weelrate2_pre"
  Demux1/15 -> [weelrate3_pre]  "weelrate3_pre"
  Demux1/16 -> [weelrate4_pre]  "weelrate4_pre"
  [driver_steering] -> Mux2/5  "theta1"
  Demux1/17 -> [exitflag]  "exitflag"
  Demux1/18 -> [max_violation]  "max_vio"
  Demux2/1 -> Demux1/1
  Demux2/2 -> Terminator/1  "MPC_model_log_vec"

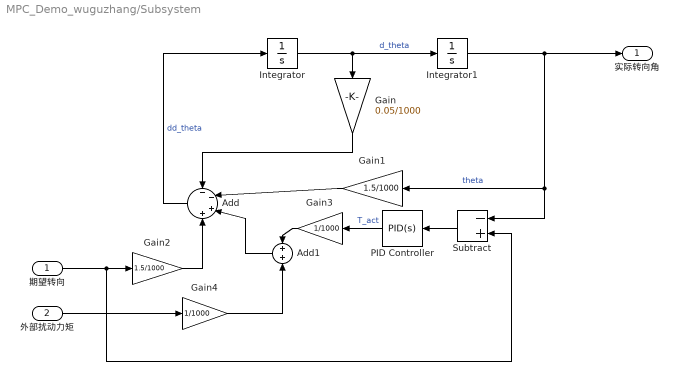
== system MPC_Demo_wuguzhang/Subsystem ==
  期望转向 : Inport
  外部扰动力矩 : Inport  Port=2
  Add : Sum  Inputs=--++
  Add1 : Sum
  Gain : Gain  Gain=0.05/1000
  Gain1 : Gain  Gain=1.5/1000
  Gain2 : Gain  Gain=1.5/1000
  Gain3 : Gain  Gain=1/1000
  Gain4 : Gain  Gain=1/1000
  Integrator : Integrator
  Integrator1 : Integrator
  PID Controller : slpidlib/PID Controller  Controller=PID  Form=Parallel  TimeDomain=Continuous-time  UseExternalTs=off  SampleTime=-1  IntegratorMethod=Forward Euler  FilterMethod=Forward Euler  ControllerParametersSource=internal  P=10000  I=100  UseKiTs=off  D=0  UseExternalDerivativeSource=off  N=100  UseFilter=on  TunerSelectOption=Transfer Function Based (PID Tuner App)  InitialConditionSource=internal  InitialConditionForIntegrator=0  InitialConditionForFilter=0  DifferentiatorICPrevScaledInput=0  ExternalReset=none  TrackingMode=off  Kt=1  LimitOutput=off  SatLimitsSource=internal  UpperSaturationLimit=inf  LowerSaturationLimit=-inf  LinearizeAsGain=on  AntiWindupMode=none  Kb=1  LimitIntegrator=off  UpperIntegratorSaturationLimit=inf  LowerIntegratorSaturationLimit=-inf  POutMin=[]  POutMax=[]  IOutMin=[]  IOutMax=[]  DOutMin=[]  DOutMax=[]  NOutMin=[]  NOutMax=[]  SumOutMin=[]  SumOutMax=[]  SaturationOutMin=[]  SaturationOutMax=[]  PParamMin=[]  PParamMax=[]  IParamMin=[]  IParamMax=[]  DParamMin=[]  DParamMax=[]  NParamMin=[]  NParamMax=[]  KbParamMin=[]  KbParamMax=[]  KtParamMin=[]  KtParamMax=[]  KbOutMin=[]  KbOutMax=[]  KtOutMin=[]  KtOutMax=[]  IntegratorOutMin=[]  IntegratorOutMax=[]  FilterOutMin=[]  FilterOutMax=[]  SumI1OutMin=[]  SumI1OutMax=[]  SumI2OutMin=[]  SumI2OutMax=[]  SumI3OutMin=[]  SumI3OutMax=[]  SumI4OutMin=[]  SumI4OutMax=[]  SumDOutMin=[]  SumDOutMax=[]  DifferentiatorOutMin=[]  DifferentiatorOutMax=[]  FilterDiffOutCoefMin=[]  FilterDiffOutCoefMax=[]  ReciprocalOutMin=[]  ReciprocalOutMax=[]  SumDenOutMin=[]  SumDenOutMax=[]  SumNumOutMin=[]  SumNumOutMax=[]  DivideOutMin=[]  DivideOutMax=[]  UdiffTsProdOutMin=[]  UdiffTsProdOutMax=[]  NTsProdOutMin=[]  NTsProdOutMax=[]  UintegralTsProdOutMin=[]  UintegralTsProdOutMax=[]  UngainTsProdOutMin=[]  UngainTsProdOutMax=[]  ClampingZeroOutDataTypeStr=Inherit: Inherit via back propagation  ClampingZeroOutMin=[]  ClampingZeroOutMax=[]  FilterDenConstantOutDataTypeStr=Inherit: Inherit via back propagation  FilterDenConstantOutMin=[]  FilterDenConstantOutMax=[]  PCopyOutDataTypeStr=Inherit: Inherit via back propagation  PCopyOutMin=[]  PCopyOutMax=[]  NCopyOutDataTypeStr=Inherit: Inherit via back propagation  NCopyOutMin=[]  NCopyOutMax=[]  IntegratorContinuousStateAttributes=''  IntegratorStateMustResolveToSignalObject=off  IntegratorRTWStateStorageClass=Auto  FilterContinuousStateAttributes=''  FilterStateMustResolveToSignalObject=off  FilterRTWStateStorageClass=Auto  ParallelPVariant=InternalParameters  IdealPVariant=Disabled  IVariant=InternalParameters  DVariant=InternalParameters  IntegratorVariant=Continuous  SatVariant=Disabled  AWVariant=Passthrough  PCopyVariant=Disabled  TRVariant=Disabled  FdbkBlocksVariant=Forward  IdealPFdbkVariant=Disabled  SatFdbkVariant=Disabled  DerivativeFilterVariant=ContFilter  NVariant=InternalParameters  NCopyVariant=Disabled  FilterICVariant=InternalICsFilter  IntegratorICVariant=InternalICs  ExternalResetVariant=Disabled  TRSumVariant=Passthrough  SumFdbkVariant=Disabled  SumVariant=Sum_PID  TsampFilterVariant=InternalTs  TsampNgainVariant=Passthrough  TsampIntegralVariant=Disabled_SignalSpec  ExternalSaturationOutDataTypeStr=Inherit: Same as second input  DerivativeSourceVariant=ErrorSignal
  Subtract : Sum  Inputs=-+
  实际转向角 : Outport
  wires:
  期望转向/1 -> Subtract/2, Gain2/1
  Gain4/1 -> Add1/2
  Integrator/1 -> Integrator1/1, Gain/1  "d_theta"
  Integrator1/1 -> 实际转向角/1, Subtract/1, Gain1/1  "theta"
  外部扰动力矩/1 -> Gain4/1
  Subtract/1 -> PID Controller/1
  Gain3/1 -> Add1/1
  Gain2/1 -> Add/4
  Add1/1 -> Add/3
  Add/1 -> Integrator/1  "dd_theta"
  Gain/1 -> Add/1
  PID Controller/1 -> Gain3/1  "T_act"
  Gain1/1 -> Add/2

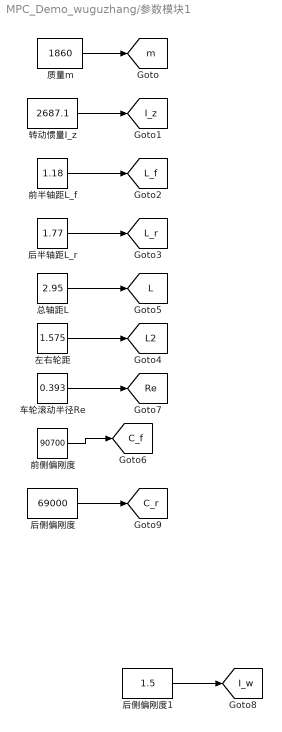
== system MPC_Demo_wuguzhang/参数模块1 ==
  前侧偏刚度 : Constant  Value=90700
  前半轴距L_f : Constant  Value=1.18
  后侧偏刚度 : Constant  Value=69000
  后侧偏刚度1 : Constant  Value=1.5
  后半轴距L_r : Constant  Value=1.77
  左右轮距 : Constant  Value=1.575
  总轴距L : Constant  Value=2.95
  质量m : Constant  Value=1860
  车轮滚动半径Re : Constant  Value=0.393
  转动惯量I_z : Constant  Value=2687.1
  tag scope: C_f=global, C_r=global, I_w=global, I_z=global, L2=global, L=global, L_f=global, L_r=global, Re=global, m=global
  wires:
  后半轴距L_r/1 -> [L_r]
  总轴距L/1 -> [L]
  车轮滚动半径Re/1 -> [Re]
  前半轴距L_f/1 -> [L_f]
  左右轮距/1 -> [L2]
  质量m/1 -> [m]
  转动惯量I_z/1 -> [I_z]
  后侧偏刚度/1 -> [C_r]
  前侧偏刚度/1 -> [C_f]
  后侧偏刚度1/1 -> [I_w]

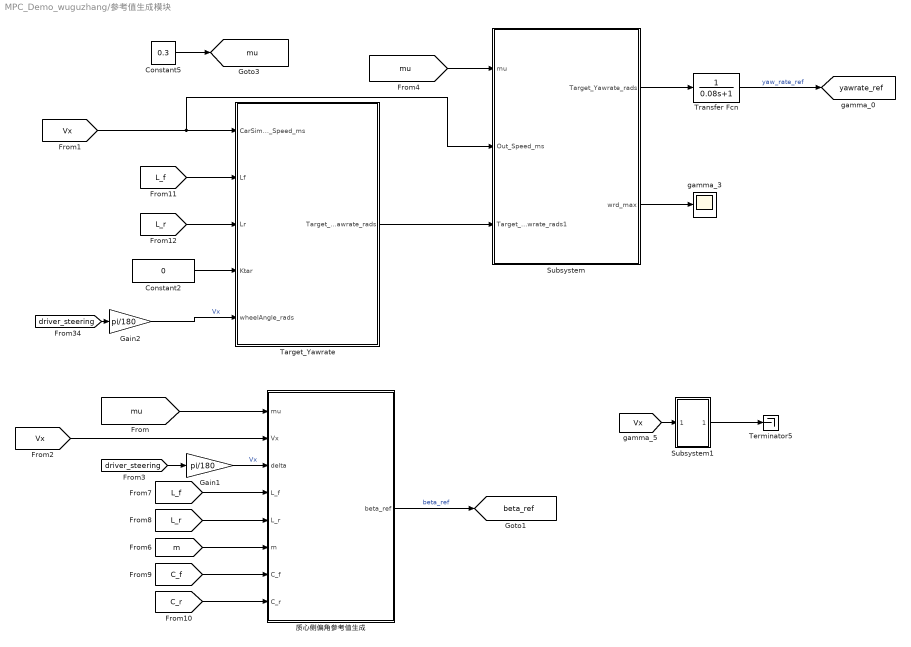
== system MPC_Demo_wuguzhang/参考值生成模块 ==
  Constant2 : Constant  Value=0
  Constant5 : Constant  Value=0.3
  Gain1 : Gain  Gain=pi/180
  Gain2 : Gain  Gain=pi/180
  Subsystem : Subsystem
  Subsystem1 : Subsystem
  Target_Yawrate : Subsystem
  Terminator5 : Terminator
  Transfer Fcn : TransferFcn  Denominator=[0.08 1]
  gamma_3 : Scope
  质心侧偏角参考值生成 : MATLAB Function  TreatAsAtomicUnit=on
  tag scope: beta_ref=global, mu=global, yawrate_ref=global
  wires:
  Target_Yawrate/1(Target_Yawrate_rads) -> Subsystem/3(Target_Yawrate_rads1)
  Subsystem/2(wrd_max) -> gamma_3/1
  [Vx] -> Subsystem/2(Out_Speed_ms), Target_Yawrate/1(CarSimOut_Speed_ms)
  [L_f] -> Target_Yawrate/2(Lf)
  [L_r] -> Target_Yawrate/3(Lr)
  [driver_steering] -> Gain2/1
  Constant2/1 -> Target_Yawrate/4(Ktar)
  Subsystem/1(Target_Yawrate_rads) -> Transfer Fcn/1
  Transfer Fcn/1 -> [yawrate_ref]  "yaw_rate_ref"
  [Vx] -> 质心侧偏角参考值生成/2(Vx)
  [driver_steering] -> Gain1/1
  质心侧偏角参考值生成/1(beta_ref) -> [beta_ref]  "beta_ref"
  [mu] -> Subsystem/1(mu)
  [mu] -> 质心侧偏角参考值生成/1(mu)
  [Vx] -> Subsystem1/1(In1)
  Subsystem1/1(Out1) -> Terminator5/1
  [m] -> 质心侧偏角参考值生成/6(m)
  [L_f] -> 质心侧偏角参考值生成/4(L_f)
  [L_r] -> 质心侧偏角参考值生成/5(L_r)
  [C_f] -> 质心侧偏角参考值生成/7(C_f)
  [C_r] -> 质心侧偏角参考值生成/8(C_r)
  Constant5/1 -> [mu]
  Gain1/1 -> 质心侧偏角参考值生成/3(delta)  "Vx"
  Gain2/1 -> Target_Yawrate/5(wheelAngle_rads)  "Vx"

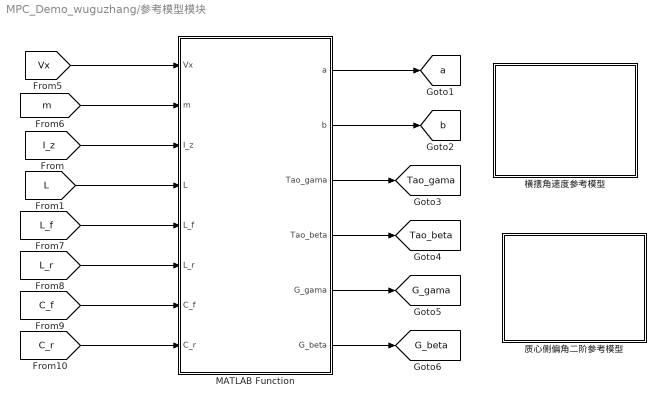
== system MPC_Demo_wuguzhang/参考模型模块 ==
  MATLAB Function : MATLAB Function  TreatAsAtomicUnit=on
  横摆角速度参考模型 : Subsystem
  质心侧偏角二阶参考模型 : Subsystem
  tag scope: G_beta=global, G_gama=global, Tao_beta=global, Tao_gama=global, a=global, b=global
  wires:
  [Vx] -> MATLAB Function/1(Vx)
  MATLAB Function/1(a) -> [a]
  MATLAB Function/2(b) -> [b]
  MATLAB Function/3(Tao_gama) -> [Tao_gama]
  MATLAB Function/4(Tao_beta) -> [Tao_beta]
  MATLAB Function/5(G_gama) -> [G_gama]
  MATLAB Function/6(G_beta) -> [G_beta]
  [m] -> MATLAB Function/2(m)
  [L_f] -> MATLAB Function/5(L_f)
  [L_r] -> MATLAB Function/6(L_r)
  [C_f] -> MATLAB Function/7(C_f)
  [C_r] -> MATLAB Function/8(C_r)
  [I_z] -> MATLAB Function/3(I_z)
  [L] -> MATLAB Function/4(L)

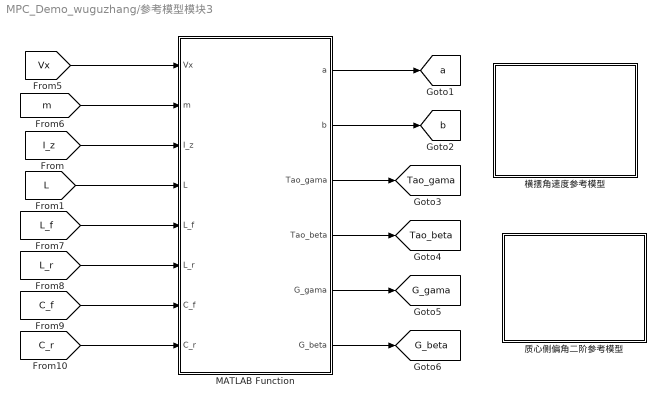
== system MPC_Demo_wuguzhang/参考模型模块3 ==
  MATLAB Function : MATLAB Function  TreatAsAtomicUnit=on
  横摆角速度参考模型 : Subsystem
  质心侧偏角二阶参考模型 : Subsystem
  tag scope: G_beta=global, G_gama=global, Tao_beta=global, Tao_gama=global, a=global, b=global
  wires:
  [Vx] -> MATLAB Function/1(Vx)
  MATLAB Function/1(a) -> [a]
  MATLAB Function/2(b) -> [b]
  MATLAB Function/3(Tao_gama) -> [Tao_gama]
  MATLAB Function/4(Tao_beta) -> [Tao_beta]
  MATLAB Function/5(G_gama) -> [G_gama]
  MATLAB Function/6(G_beta) -> [G_beta]
  [m] -> MATLAB Function/2(m)
  [L_f] -> MATLAB Function/5(L_f)
  [L_r] -> MATLAB Function/6(L_r)
  [C_f] -> MATLAB Function/7(C_f)
  [C_r] -> MATLAB Function/8(C_r)
  [I_z] -> MATLAB Function/3(I_z)
  [L] -> MATLAB Function/4(L)

== system MPC_Demo_wuguzhang/参考值生成模块/Subsystem ==
  mu : Inport
  Out_Speed_ms : Inport  Port=2
  Target_Yawrate_rads1 : Inport  Port=3
  MATLAB Function : MATLAB Function  TreatAsAtomicUnit=on
  Target_Yawrate_rads : Outport
  wrd_max : Outport  Port=2
  wires:
  Out_Speed_ms/1 -> MATLAB Function/2(vx)
  MATLAB Function/2(wrd) -> Target_Yawrate_rads/1
  mu/1 -> MATLAB Function/1(mu)
  MATLAB Function/1(wrd_max) -> wrd_max/1
  Target_Yawrate_rads1/1 -> MATLAB Function/3(wrd1)

== system MPC_Demo_wuguzhang/参考值生成模块/Subsystem1 ==
  In1 : Inport
  Constant : Constant  Value=0.01
  Ramp : simulink/Sources/Ramp  slope=1  start=0  InitialOutput=0
  Switch : Switch  Threshold=0.01  SaturateOnIntegerOverflow=off  InputSameDT=off
  Out1 : Outport
  wires:
  Switch/1 -> Out1/1
  Constant/1 -> Switch/3
  In1/1 -> Switch/1
  Ramp/1 -> Switch/2

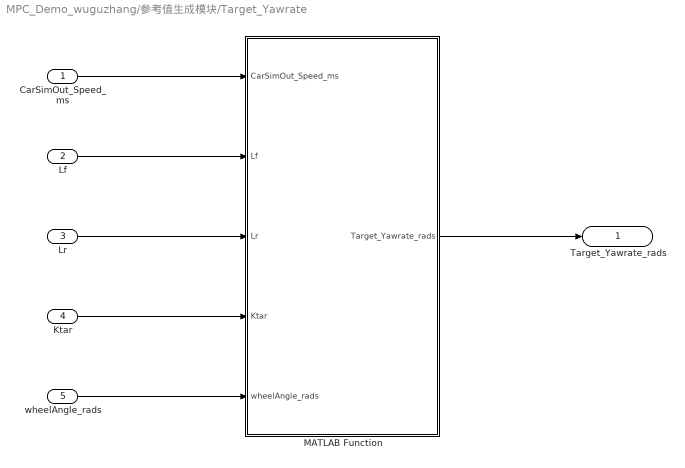
== system MPC_Demo_wuguzhang/参考值生成模块/Target_Yawrate ==
  CarSimOut_Speed_ms : Inport
  Lf : Inport  Port=2
  Lr : Inport  Port=3
  Ktar : Inport  Port=4
  wheelAngle_rads : Inport  Port=5
  MATLAB Function : MATLAB Function  TreatAsAtomicUnit=on
  Target_Yawrate_rads : Outport
  wires:
  CarSimOut_Speed_ms/1 -> MATLAB Function/1(CarSimOut_Speed_ms)
  Lf/1 -> MATLAB Function/2(Lf)
  Lr/1 -> MATLAB Function/3(Lr)
  Ktar/1 -> MATLAB Function/4(Ktar)
  wheelAngle_rads/1 -> MATLAB Function/5(wheelAngle_rads)
  MATLAB Function/1(Target_Yawrate_rads) -> Target_Yawrate_rads/1

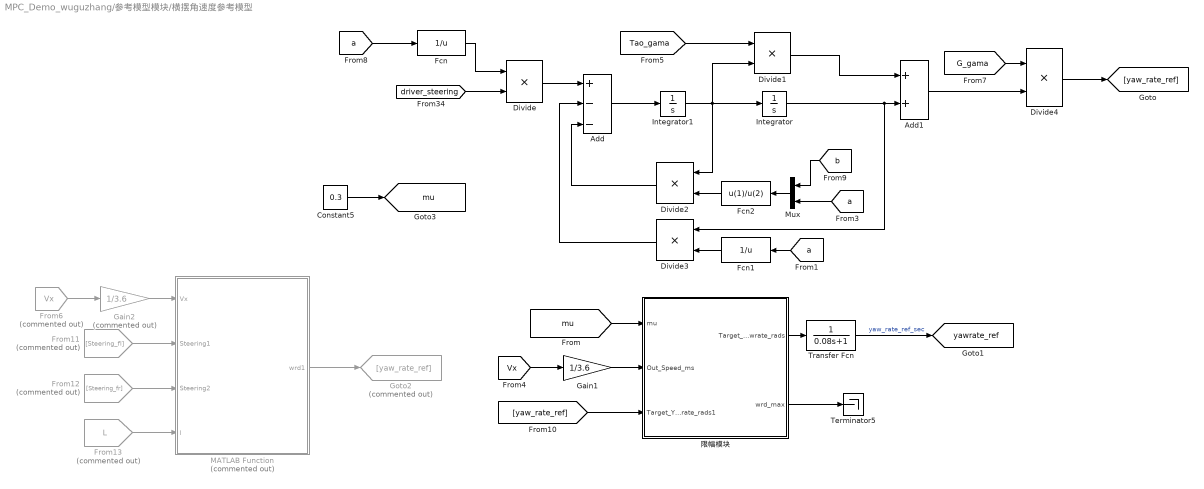
== system MPC_Demo_wuguzhang/参考模型模块/横摆角速度参考模型 ==
  Add : Sum  Inputs=+--
  Add1 : Sum
  Constant5 : Constant  Value=0.3
  Divide{,1..4} (5 alike) : Product  Inputs=**
  Fcn : Fcn  Expr=1/u
  Fcn1 : Fcn  Expr=1/u
  Fcn2 : Fcn  Expr=u(1)/u(2)
  From11 : From  Commented=on  GotoTag=Steering_fl  TagVisibility=global
  From12 : From  Commented=on  GotoTag=Steering_fr  TagVisibility=global
  From13 : From  Commented=on  GotoTag=L  TagVisibility=global
  From6 : From  Commented=on  GotoTag=Vx  TagVisibility=global
  Gain1 : Gain  Gain=1/3.6
  Gain2 : Gain  Commented=on  Gain=1/3.6
  Goto2 : Goto  Commented=on  GotoTag=yaw_rate_ref
  Integrator : Integrator
  Integrator1 : Integrator
  MATLAB Function : MATLAB Function  Commented=on  TreatAsAtomicUnit=on
  Mux : Mux  Inputs=2
  Terminator5 : Terminator
  Transfer Fcn : TransferFcn  Denominator=[0.08 1]
  限幅模块 : Subsystem
  tag scope: mu=global, yawrate_ref=global
  wires:
  Integrator/1 -> Divide3/1, Add1/2
  [G_gama] -> Divide4/1
  Add1/1 -> Divide4/2
  [Tao_gama] -> Divide1/1
  Fcn/1 -> Divide/1
  Divide4/1 -> [yaw_rate_ref]
  Fcn1/1 -> Divide3/2
  Divide2/1 -> Add/3
  Divide3/1 -> Add/2
  Fcn2/1 -> Divide2/2
  Divide/1 -> Add/1
  Divide1/1 -> Add1/1
  Integrator1/1 -> Divide2/1, Divide1/2, Integrator/1
  [driver_steering] -> Divide/2
  [a] -> Fcn/1
  [a] -> Fcn1/1
  Mux/1 -> Fcn2/1
  [b] -> Mux/1
  [a] -> Mux/2
  [mu] -> 限幅模块/1(mu)
  [Vx] -> Gain1/1
  Gain1/1 -> 限幅模块/2(Out_Speed_ms)
  [yaw_rate_ref] -> 限幅模块/3(Target_Yawrate_rads1)
  限幅模块/1(Target_Yawrate_rads) -> Transfer Fcn/1
  Transfer Fcn/1 -> [yawrate_ref]  "yaw_rate_ref_sec"
  限幅模块/2(wrd_max) -> Terminator5/1
  MATLAB Function/1(wrd1) -> Goto2/1
  From11/1 -> MATLAB Function/2(Steering1)
  From12/1 -> MATLAB Function/3(Steering2)
  From13/1 -> MATLAB Function/4(l)
  From6/1 -> Gain2/1
  Gain2/1 -> MATLAB Function/1(Vx)
  Constant5/1 -> [mu]
  Add/1 -> Integrator1/1

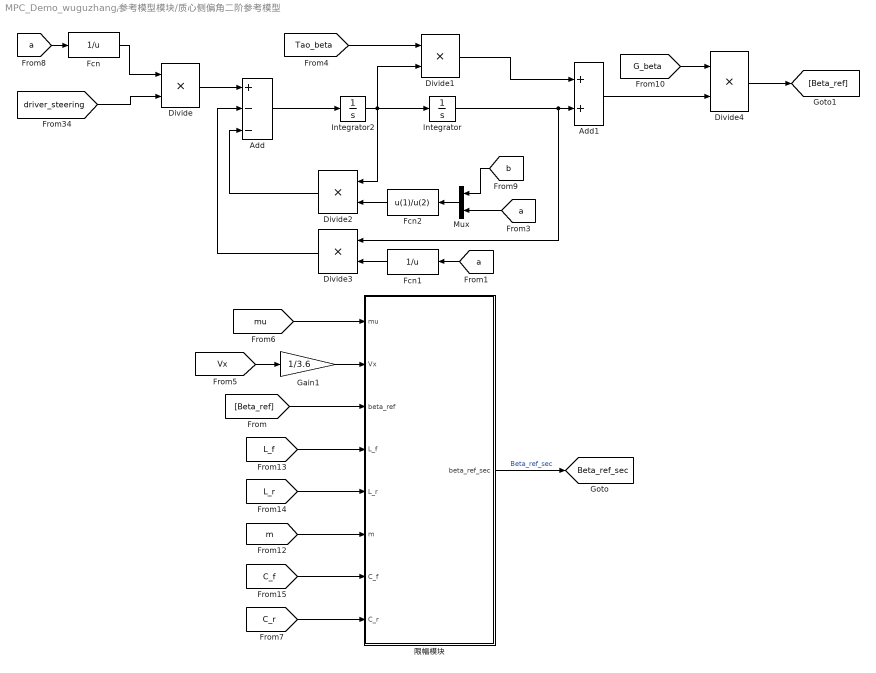
== system MPC_Demo_wuguzhang/参考模型模块/质心侧偏角二阶参考模型 ==
  Add : Sum  Inputs=+--
  Add1 : Sum
  Divide{,1..4} (5 alike) : Product  Inputs=**
  Fcn : Fcn  Expr=1/u
  Fcn1 : Fcn  Expr=1/u
  Fcn2 : Fcn  Expr=u(1)/u(2)
  Gain1 : Gain  Gain=1/3.6
  Integrator : Integrator
  Integrator2 : Integrator
  Mux : Mux  Inputs=2
  限幅模块 : MATLAB Function  TreatAsAtomicUnit=on
  tag scope: Beta_ref_sec=global
  wires:
  [a] -> Mux/2
  [b] -> Mux/1
  Mux/1 -> Fcn2/1
  [a] -> Fcn1/1
  [a] -> Fcn/1
  [driver_steering] -> Divide/2
  Integrator2/1 -> Integrator/1, Divide1/2, Divide2/1
  Divide1/1 -> Add1/1
  Divide/1 -> Add/1
  Fcn2/1 -> Divide2/2
  Divide3/1 -> Add/2
  Divide2/1 -> Add/3
  Fcn1/1 -> Divide3/2
  Divide4/1 -> [Beta_ref]
  Fcn/1 -> Divide/1
  [Tao_beta] -> Divide1/1
  Add1/1 -> Divide4/2
  [G_beta] -> Divide4/1
  Integrator/1 -> Add1/2, Divide3/1
  [mu] -> 限幅模块/1(mu)
  限幅模块/1(beta_ref_sec) -> [Beta_ref_sec]  "Beta_ref_sec"
  [Beta_ref] -> 限幅模块/3(beta_ref)
  [Vx] -> Gain1/1
  Gain1/1 -> 限幅模块/2(Vx)
  Add/1 -> Integrator2/1
  [m] -> 限幅模块/6(m)
  [L_f] -> 限幅模块/4(L_f)
  [L_r] -> 限幅模块/5(L_r)
  [C_f] -> 限幅模块/7(C_f)
  [C_r] -> 限幅模块/8(C_r)

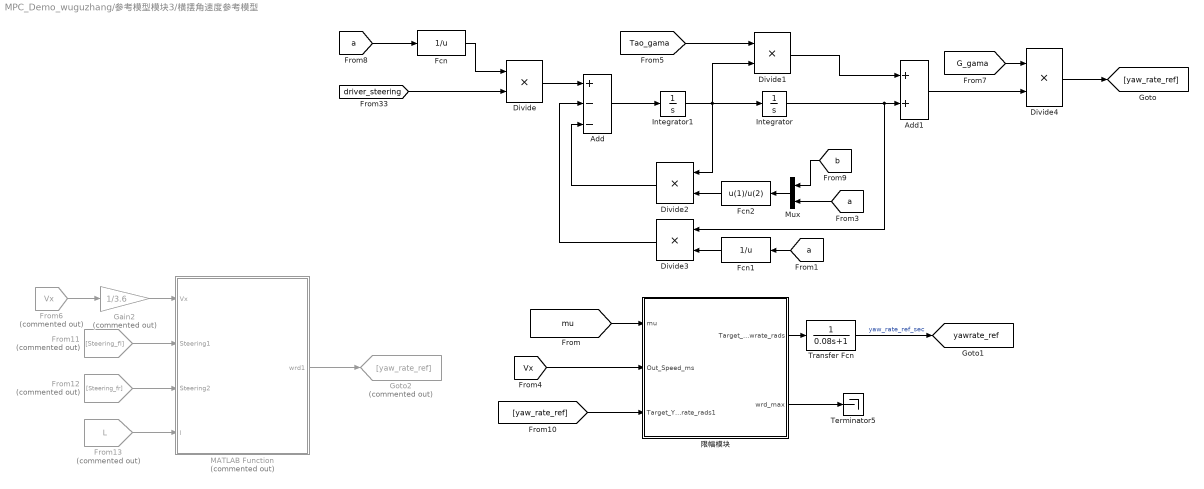
== system MPC_Demo_wuguzhang/参考模型模块3/横摆角速度参考模型 ==
  Add : Sum  Inputs=+--
  Add1 : Sum
  Divide{,1..4} (5 alike) : Product  Inputs=**
  Fcn : Fcn  Expr=1/u
  Fcn1 : Fcn  Expr=1/u
  Fcn2 : Fcn  Expr=u(1)/u(2)
  From11 : From  Commented=on  GotoTag=Steering_fl  TagVisibility=global
  From12 : From  Commented=on  GotoTag=Steering_fr  TagVisibility=global
  From13 : From  Commented=on  GotoTag=L  TagVisibility=global
  From6 : From  Commented=on  GotoTag=Vx  TagVisibility=global
  Gain2 : Gain  Commented=on  Gain=1/3.6
  Goto2 : Goto  Commented=on  GotoTag=yaw_rate_ref
  Integrator : Integrator
  Integrator1 : Integrator
  MATLAB Function : MATLAB Function  Commented=on  TreatAsAtomicUnit=on
  Mux : Mux  Inputs=2
  Terminator5 : Terminator
  Transfer Fcn : TransferFcn  Denominator=[0.08 1]
  限幅模块 : Subsystem
  tag scope: yawrate_ref=global
  wires:
  Integrator/1 -> Divide3/1, Add1/2
  [G_gama] -> Divide4/1
  Add1/1 -> Divide4/2
  [Tao_gama] -> Divide1/1
  Fcn/1 -> Divide/1
  Divide4/1 -> [yaw_rate_ref]
  Fcn1/1 -> Divide3/2
  Divide2/1 -> Add/3
  Divide3/1 -> Add/2
  Fcn2/1 -> Divide2/2
  Divide/1 -> Add/1
  Divide1/1 -> Add1/1
  Integrator1/1 -> Divide2/1, Divide1/2, Integrator/1
  [a] -> Fcn/1
  [a] -> Fcn1/1
  Mux/1 -> Fcn2/1
  [b] -> Mux/1
  [a] -> Mux/2
  [mu] -> 限幅模块/1(mu)
  [Vx] -> 限幅模块/2(Out_Speed_ms)
  [yaw_rate_ref] -> 限幅模块/3(Target_Yawrate_rads1)
  限幅模块/1(Target_Yawrate_rads) -> Transfer Fcn/1
  Transfer Fcn/1 -> [yawrate_ref]  "yaw_rate_ref_sec"
  限幅模块/2(wrd_max) -> Terminator5/1
  MATLAB Function/1(wrd1) -> Goto2/1
  From11/1 -> MATLAB Function/2(Steering1)
  From12/1 -> MATLAB Function/3(Steering2)
  From13/1 -> MATLAB Function/4(l)
  From6/1 -> Gain2/1
  Gain2/1 -> MATLAB Function/1(Vx)
  Add/1 -> Integrator1/1
  [driver_steering] -> Divide/2

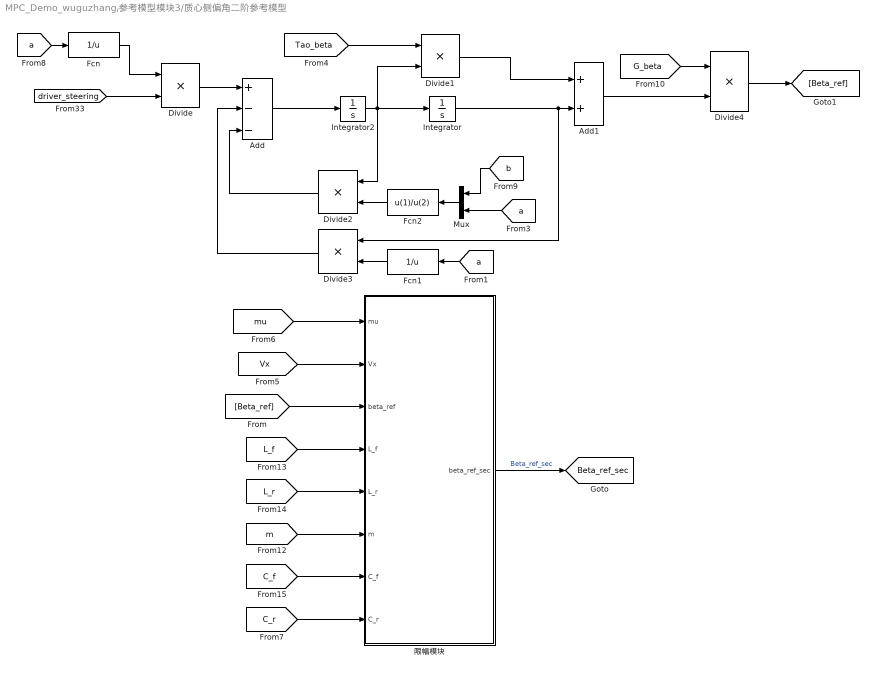
== system MPC_Demo_wuguzhang/参考模型模块3/质心侧偏角二阶参考模型 ==
  Add : Sum  Inputs=+--
  Add1 : Sum
  Divide{,1..4} (5 alike) : Product  Inputs=**
  Fcn : Fcn  Expr=1/u
  Fcn1 : Fcn  Expr=1/u
  Fcn2 : Fcn  Expr=u(1)/u(2)
  Integrator : Integrator
  Integrator2 : Integrator
  Mux : Mux  Inputs=2
  限幅模块 : MATLAB Function  TreatAsAtomicUnit=on
  tag scope: Beta_ref_sec=global
  wires:
  [a] -> Mux/2
  [b] -> Mux/1
  Mux/1 -> Fcn2/1
  [a] -> Fcn1/1
  [a] -> Fcn/1
  Integrator2/1 -> Integrator/1, Divide1/2, Divide2/1
  Divide1/1 -> Add1/1
  Divide/1 -> Add/1
  Fcn2/1 -> Divide2/2
  Divide3/1 -> Add/2
  Divide2/1 -> Add/3
  Fcn1/1 -> Divide3/2
  Divide4/1 -> [Beta_ref]
  Fcn/1 -> Divide/1
  [Tao_beta] -> Divide1/1
  Add1/1 -> Divide4/2
  [G_beta] -> Divide4/1
  Integrator/1 -> Add1/2, Divide3/1
  [mu] -> 限幅模块/1(mu)
  限幅模块/1(beta_ref_sec) -> [Beta_ref_sec]  "Beta_ref_sec"
  [Beta_ref] -> 限幅模块/3(beta_ref)
  [Vx] -> 限幅模块/2(Vx)
  Add/1 -> Integrator2/1
  [m] -> 限幅模块/6(m)
  [L_f] -> 限幅模块/4(L_f)
  [L_r] -> 限幅模块/5(L_r)
  [C_f] -> 限幅模块/7(C_f)
  [C_r] -> 限幅模块/8(C_r)
  [driver_steering] -> Divide/2

== system MPC_Demo_wuguzhang/参考模型模块/横摆角速度参考模型/限幅模块 ==
  mu : Inport
  Out_Speed_ms : Inport  Port=2
  Target_Yawrate_rads1 : Inport  Port=3
  MATLAB Function : MATLAB Function  TreatAsAtomicUnit=on
  Target_Yawrate_rads : Outport
  wrd_max : Outport  Port=2
  wires:
  Out_Speed_ms/1 -> MATLAB Function/2(vx)
  MATLAB Function/2(wrd) -> Target_Yawrate_rads/1
  mu/1 -> MATLAB Function/1(mu)
  MATLAB Function/1(wrd_max) -> wrd_max/1
  Target_Yawrate_rads1/1 -> MATLAB Function/3(wrd1)

== system MPC_Demo_wuguzhang/参考模型模块3/横摆角速度参考模型/限幅模块 ==
  mu : Inport
  Out_Speed_ms : Inport  Port=2
  Target_Yawrate_rads1 : Inport  Port=3
  MATLAB Function : MATLAB Function  TreatAsAtomicUnit=on
  Target_Yawrate_rads : Outport
  wrd_max : Outport  Port=2
  wires:
  Out_Speed_ms/1 -> MATLAB Function/2(vx)
  MATLAB Function/2(wrd) -> Target_Yawrate_rads/1
  mu/1 -> MATLAB Function/1(mu)
  MATLAB Function/1(wrd_max) -> wrd_max/1
  Target_Yawrate_rads1/1 -> MATLAB Function/3(wrd1)

== matlab function MPC_Demo_wuguzhang/参考模型模块/横摆角速度参考模型/限幅模块/MATLAB Function ==
  data: mu input; wrd_max output; vx input; wrd1 input; wrd output
function [wrd_max,wrd]= fcn(mu,vx,wrd1)
%#eml
wrd_max=mu*9.8/(vx);


if abs(wrd1)<=abs(wrd_max)
    wrd=wrd1;
elseif wrd1>0
    wrd=abs(wrd_max);
else
    wrd=-abs(wrd_max);
end


end
